simulink model "averagebuck_juanjo"  (R2019a)
settings: Solver=FixedStepAuto  StartTime=0.0  StopTime=30  FixedStep=1e-1  RelTol=1e-3
libraries: powerlib x7, simulink x2
settings Model: Creator=Soto Porras  LastModifiedBy=juanj
settings DataIOCC: ReturnWorkspaceOutputs=off
settings DebuggingCC: ArithmeticOperatorsInVariantConditions=warning

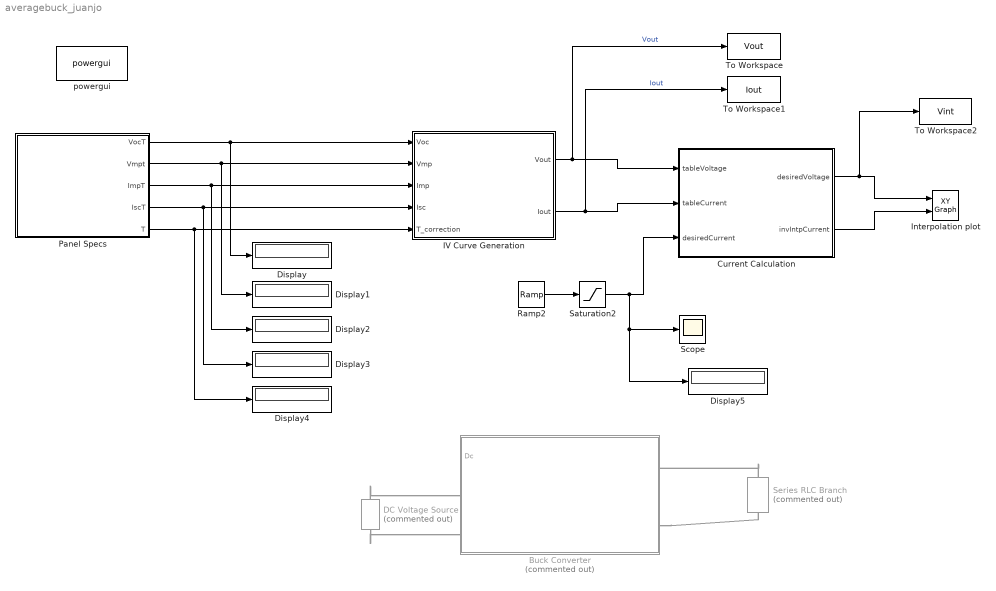
== system averagebuck_juanjo ==
  Buck Converter : Subsystem  Commented=on
  Current Calculation : MATLAB Function  TreatAsAtomicUnit=on
  DC Voltage Source : powerlib/Electrical Sources/DC Voltage Source  Commented=on  Amplitude=15  Measurements=None
      settings: SourceProductName=Simscape Electrical
  Display{,1..5} (6 alike) : Display
  IV Curve Generation : Subsystem  mask(Panel I-V Curve Calculation){ValueVocComp=0.0062, ValueVmpComp=0.0067}
      mask prompts: ValueVocComp "Voc Temperature Correction (V)"; ValueVmpComp "Vmp Temperature Correction (V)"
      mask help:
      | This module calculates the panel IV curve using the next panel parameters:
      | 1. Voc
      | 2. Vmp
      | 3. Imp
      | 4. Isc
      |
      | It applies:
      | 1. Correction to current parameters (Isc and Imp) using a pseudo cosine that varies depending on the angle of the perpendicular CubeSat face and the sun's incident radiation.
      | 2. Correction to voltage parameters (Voc and Vmp) using the panel datasheet voltage losses, given in V by the user.
      mask TypeOptions ValueVocComp: Voc_comp/Value
      mask TypeOptions ValueVmpComp: Vmp_comp/Value
      mask Display: image('IV_curve.png');
  Interpolation plot : simulink/Sinks/XY Graph  xmin=0  xmax=6  ymin=0  ymax=2  st=-1
  Panel Specs : Subsystem  mask(Solar Panel Specifications){Voc=2.690, Vmp=2.409, Imp=0.5029, Isc=0.5196, Temp=28, SerialGain=2, ParallelGain=3}
      mask prompts: Temp "T°"; SerialGain "Serial"; ParallelGain "Parallel"
      mask help: Inputs solar panel electrical specifications, temperature and array distribution.
      mask TypeOptions Voc: Voc/Value
      mask TypeOptions Vmp: Vmp/Value
      mask TypeOptions Imp: Imp/Value
      mask TypeOptions Isc: Isc/Value
      mask TypeOptions Temp: T°/Value
      mask TypeOptions SerialGain: Gain/Gain | Gain1/Gain
      mask TypeOptions ParallelGain: Gain2/Gain | Gain3/Gain
      mask DialogControl Container3 Prompt: Panel Array
      mask Display: image('solar_panel.png');
  Ramp2 : simulink/Sources/Ramp  slope=0.051967  start=0  InitialOutput=0
  Saturation2 : Saturate  UpperLimit=1.5603  LowerLimit=0
  Scope : Scope
  Series RLC Branch : powerlib/Elements/Series RLC Branch  Commented=on  LConnTagsString=__new0  RConnTagsString=__new0  BranchType=R  Resistance=5  Inductance=1e-3  SetiL0=off  InitialCurrent=0  Capacitance=1e-6  Setx0=off  InitialVoltage=0  Measurements=None
      settings: SourceProductName=Simscape Electrical
  To Workspace : ToWorkspace  VariableName=Vout  SaveFormat=Structure With Time  SampleTime=-1
  To Workspace1 : ToWorkspace  VariableName=Iout  SaveFormat=Structure With Time  SampleTime=-1
  To Workspace2 : ToWorkspace  VariableName=Vint  SaveFormat=Structure With Time  SampleTime=-1
  powergui : powerlib/powergui  Priority=1  SimulationMode=Continuous  SampleTime=50e-6  frequency=60  Iterations=50  frequencyindice=0  Pbase=100e6  ErrMax=1e-4  UnitsV=kV  UnitsW=MW  buscounter=0  FunctionMessages=off  echomessages=off  EnableUseOfTLC=off  CurrentSourceSwitches=off  DisableSnubberDevices=off  DisableRonSwitches=off  DisableVfSwitches=off  DisplayEquations=off  AutomaticDiscreteSolvers=off  SolverType=Tustin/Backward Euler (TBE)  Interpol=off  ExternalGateDelay=off  methode=off  Ts=100  x0status=blocks  SPID=on  SwTol=0  HookPort=off  NonlinearTolerance=0  nMaxIteration=15  ContinueOnMaxIteration=off  RestoreLinks=warning  ResistiveCurrentMeasurement=off  Frange=[0:2:500]  Ylog=off  Xlog=on  ShowGrid=off  save=off  variable=ZData  structure=0  ZoomFFT=off  StartTime=0.0  cycles=1  DisplayStyle=1  fundamental=60  FreqAxis=off  MaxFrequency=1000  frequencyindicesteady=1  RmsSteady=1  display=off
      settings: SourceProductName=Simscape Electrical
  wires:
  Panel Specs/1(VocT) -> IV Curve Generation/1(Voc), Display/1
  Panel Specs/2(Vmpt) -> IV Curve Generation/2(Vmp), Display1/1
  Panel Specs/3(ImpT) -> IV Curve Generation/3(Imp), Display2/1
  Panel Specs/4(IscT) -> IV Curve Generation/4(Isc), Display3/1
  Panel Specs/5(T) -> IV Curve Generation/5(T_correction), Display4/1
  Ramp2/1 -> Saturation2/1
  IV Curve Generation/1(Vout) -> To Workspace/1, Current Calculation/1(tableVoltage)  "Vout"
  IV Curve Generation/2(Iout) -> To Workspace1/1, Current Calculation/2(tableCurrent)  "Iout"
  Saturation2/1 -> Display5/1, Scope/1, Current Calculation/3(desiredCurrent)
  Current Calculation/2(invIntpCurrent) -> Interpolation plot/2
  Current Calculation/1(desiredVoltage) -> To Workspace2/1, Interpolation plot/1
  connections:
  DC Voltage Source/RConn1 -- Buck Converter/LConn1
  DC Voltage Source/LConn1 -- Buck Converter/LConn2
  Series RLC Branch/LConn1 -- Buck Converter/RConn1
  Buck Converter/RConn2 -- Series RLC Branch/RConn1

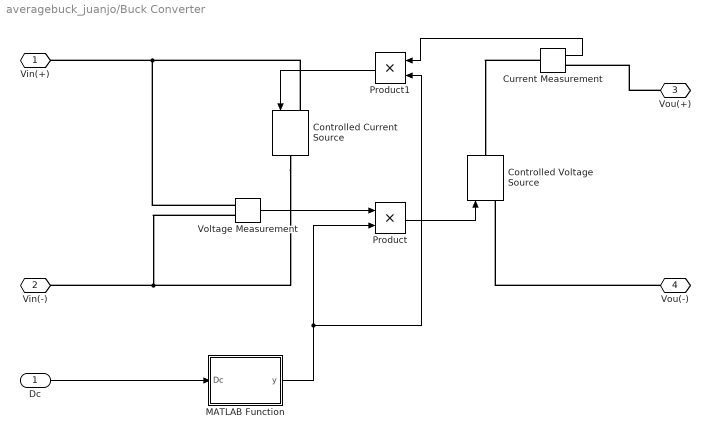
== system averagebuck_juanjo/Buck Converter ==
  Dc : Inport
  Controlled Current Source : powerlib/Electrical Sources/Controlled Current Source  Initialize=off  Source_Type=DC  Amplitude=0  Phase=0  Frequency=0  Measurements=None
      settings: SourceProductName=Simscape Electrical
  Controlled Voltage Source : powerlib/Electrical Sources/Controlled Voltage Source  Initialize=off  Source_Type=DC  Amplitude=0  Phase=0  Frequency=0  Measurements=None
      settings: SourceProductName=Simscape Electrical
  Current Measurement : powerlib/Measurements/Current Measurement  PhasorSimulation=off  OutputType=Complex  PSBequivalent=0
      settings: SourceProductName=Simscape Electrical
  MATLAB Function : MATLAB Function  TreatAsAtomicUnit=on
  Product : Product
  Product1 : Product
  Voltage Measurement : powerlib/Measurements/Voltage Measurement  PhasorSimulation=off  OutputType=Complex  PSBequivalent=0
      settings: SourceProductName=Simscape Electrical
  Vin(+) : PMIOPort  Side=Left
  Vin(-) : PMIOPort  Port=2  Side=Left
  Vou(+) : PMIOPort  Port=3  Side=Right
  Vou(-) : PMIOPort  Port=4  Side=Right
  wires:
  Product/1 -> Controlled Voltage Source/1
  Current Measurement/1 -> Product1/1
  Product1/1 -> Controlled Current Source/1
  MATLAB Function/1(y) -> Product1/2, Product/2
  Voltage Measurement/1 -> Product/1
  Dc/1 -> MATLAB Function/1(Dc)
  connections:
  Controlled Current Source/RConn1 -- Voltage Measurement/LConn2 -- Vin(-)/RConn1
  Vou(-)/RConn1 -- Controlled Voltage Source/LConn1
  Current Measurement/LConn1 -- Controlled Voltage Source/RConn1
  Controlled Current Source/LConn1 -- Voltage Measurement/LConn1 -- Vin(+)/RConn1
  Vou(+)/RConn1 -- Current Measurement/RConn1

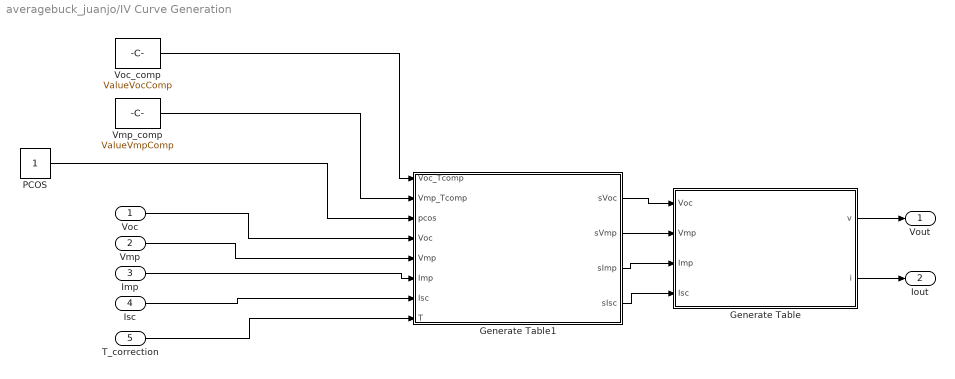
== system averagebuck_juanjo/IV Curve Generation ==
  Voc : Inport
  Vmp : Inport  Port=2
  Imp : Inport  Port=3
  Isc : Inport  Port=4
  T_correction : Inport  Port=5
  Generate Table : MATLAB Function  TreatAsAtomicUnit=on
  Generate Table1 : MATLAB Function  TreatAsAtomicUnit=on
  PCOS : Constant
  Vmp_comp : Constant  Value=ValueVmpComp
  Voc_comp : Constant  Value=ValueVocComp
  Vout : Outport
  Iout : Outport  Port=2
  wires:
  Isc/1 -> Generate Table1/7(Isc)
  Generate Table1/4(sIsc) -> Generate Table/4(Isc)
  Voc_comp/1 -> Generate Table1/1(Voc_Tcomp)
  Generate Table/1(v) -> Vout/1
  T_correction/1 -> Generate Table1/8(T)
  Generate Table1/2(sVmp) -> Generate Table/2(Vmp)
  Voc/1 -> Generate Table1/4(Voc)
  PCOS/1 -> Generate Table1/3(pcos)
  Generate Table1/3(sImp) -> Generate Table/3(Imp)
  Imp/1 -> Generate Table1/6(Imp)
  Generate Table1/1(sVoc) -> Generate Table/1(Voc)
  Vmp/1 -> Generate Table1/5(Vmp)
  Generate Table/2(i) -> Iout/1
  Vmp_comp/1 -> Generate Table1/2(Vmp_Tcomp)

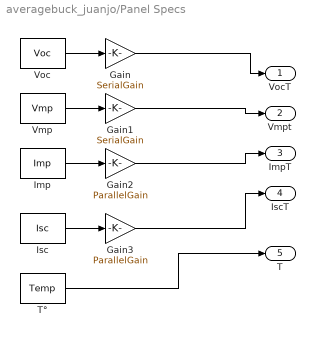
== system averagebuck_juanjo/Panel Specs ==
  Gain : Gain  Gain=SerialGain
  Gain1 : Gain  Gain=SerialGain
  Gain2 : Gain  Gain=ParallelGain
  Gain3 : Gain  Gain=ParallelGain
  Imp : Constant  Value=Imp
  Isc : Constant  Value=Isc
  T° : Constant  Value=Temp
  Vmp : Constant  Value=Vmp
  Voc : Constant  Value=Voc
  VocT : Outport
  Vmpt : Outport  Port=2
  ImpT : Outport  Port=3
  IscT : Outport  Port=4
  T : Outport  Port=5
  wires:
  Isc/1 -> Gain3/1
  Vmp/1 -> Gain1/1
  Gain/1 -> VocT/1
  Imp/1 -> Gain2/1
  Gain2/1 -> ImpT/1
  Gain3/1 -> IscT/1
  Voc/1 -> Gain/1
  Gain1/1 -> Vmpt/1
  T°/1 -> T/1

== matlab function averagebuck_juanjo/Buck Converter/MATLAB Function ==
  data: Dc input; y output
function y = M(Dc)
y = Dc;

== matlab function averagebuck_juanjo/Current Calculation ==
  data: desiredVoltage output; tableVoltage input; tableCurrent input; invIntpCurrent output; desiredCurrent input
function [desiredVoltage, invIntpCurrent] = CurrentInverseInterpolation(tableVoltage, tableCurrent, desiredCurrent)
    
    % Apply inverse interpolation on ampere ramp values
    n = 1024;
    y = desiredCurrent;
    invIntpVoltageHelper = 0;
    v = 0;
    %i = 1023;
    for j = 1 : n - 1
        i = 1024 - j;
        if(desiredCurrent < tableCurrent(i))
           v = tableVoltage(i) + (tableVoltage(i+1)-tableVoltage(i))*((desiredCurrent - tableCurrent(i))/(tableCurrent(i+1) - tableCurrent(i)));
           break;
        end
    end

    
%     for i = 1 : n
%         vi = tableVoltage(i);
%         for j = 1 : n
%             if(j ~= i)
%                 vi = vi*((y-tableCurrent(j))/(tableCurrent(i) - tableCurrent(j)));
%             end
%         end
%         invIntpVoltageHelper = invIntpVoltageHelper + vi;
%     end
% 
     desiredVoltage = v;
     invIntpCurrent = desiredCurrent;
    
end

== matlab function averagebuck_juanjo/IV Curve Generation/Generate Table ==
  data: Voc input; Vmp input; Imp input; Isc input; v output; i output
function [v,i] = generate_table(Voc, Vmp, Imp, Isc)
Rs = ( Voc - Vmp ) / Imp;
a = ( Vmp * ( 1 + ( Rs*Isc ) / Voc ) + Rs*( Imp - Isc ) ) / Voc;
N = log( 2 - 2^a) / log ( Imp / Isc );
i=zeros(1024,1);
v=zeros(1024,1);
for x = 1:1024
    I = (x * Isc) / 1023.0;
    V = Voc * log( 2 - ( ( I / Isc ) ^ N ) );
    V = V / log( 2 );
    V = V - Rs * ( I - Isc );
    V = V / ( 1 + ( ( Rs * Isc) / Voc) );
    P = V * I;
    v(x) = V;
    i(x) = I;
end
v = flip(v);
i = flip(i);

== matlab function averagebuck_juanjo/IV Curve Generation/Generate Table1 ==
  data: Voc_Tcomp input; Vmp_Tcomp input; pcos input; Voc input; Vmp input; Imp input; Isc input; sVoc output; sVmp output; sImp output; sIsc output; T input
function [sVoc, sVmp, sImp, sIsc] = scalevars(Voc_Tcomp, Vmp_Tcomp, pcos, Voc, Vmp, Imp, Isc, T)
sVoc = Voc-(T*Voc_Tcomp);
sVmp = Vmp-(T*Vmp_Tcomp);
sImp = pcos * Imp;
sIsc = pcos * Isc;
